simulink model "part1_2"  (R2019b)
settings: Solver=VariableStepAuto  StartTime=0.0  StopTime=9  RelTol=1e-3
libraries: simulink x1
settings Model: Creator=wes_m  LastModifiedBy=wes_m

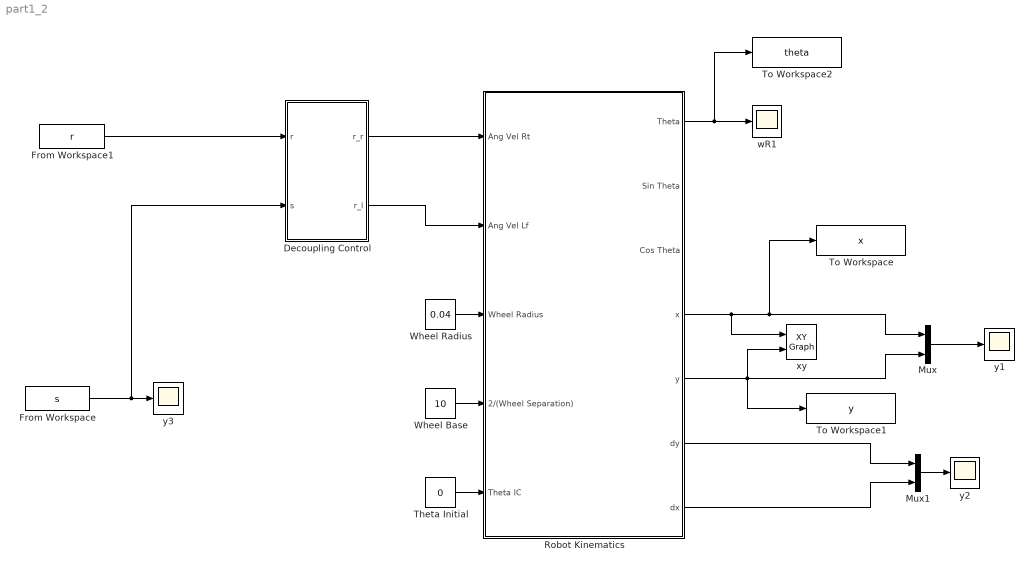
== system part1_2 ==
  Decoupling Control : Subsystem
  From Workspace : FromWorkspace  VariableName=s  SampleTime=0
  From Workspace1 : FromWorkspace  VariableName=r  SampleTime=0
  Mux : Mux  Inputs=2
  Mux1 : Mux  Inputs=2
  Robot Kinematics : Subsystem
  Theta Initial : Constant  Value=0  VectorParams1D=off  OutDataTypeStr=double
  To Workspace : ToWorkspace  VariableName=x  SampleTime=-1
  To Workspace1 : ToWorkspace  VariableName=y  SampleTime=-1
  To Workspace2 : ToWorkspace  VariableName=theta  SampleTime=-1
  Wheel Base : Constant  Value=10
  Wheel Radius : Constant  Value=0.04
  wR1 : Scope
  xy : simulink/Sinks/XY Graph  xmin=-0.1  xmax=0.5  ymin=-0.1  ymax=0.1  st=-1
  y1 : Scope
  y2 : Scope
  y3 : Scope
  wires:
  Decoupling Control/2("r_l ") -> Robot Kinematics/2(Ang Vel Lf)
  From Workspace/1 -> y3/1, Decoupling Control/2(s)
  Mux1/1 -> y2/1
  Robot Kinematics/6(dy) -> Mux1/1
  Theta Initial/1 -> Robot Kinematics/5(Theta IC)
  Decoupling Control/1(r_r) -> Robot Kinematics/1(Ang Vel Rt)
  Robot Kinematics/5(y) -> To Workspace1/1, xy/2, Mux/2
  Wheel Base/1 -> Robot Kinematics/4(2/(Wheel Separation))
  From Workspace1/1 -> Decoupling Control/1(r)
  Robot Kinematics/1(Theta) -> To Workspace2/1, wR1/1
  Robot Kinematics/4(x) -> xy/1, To Workspace/1, Mux/1
  Wheel Radius/1 -> Robot Kinematics/3(Wheel Radius)
  Mux/1 -> y1/1
  Robot Kinematics/7(dx) -> Mux1/2

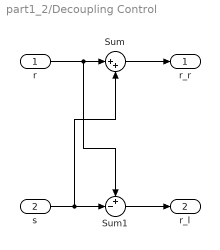
== system part1_2/Decoupling Control ==
  r : Inport
  s : Inport  Port=2
  Sum : Sum  Inputs=|++
  Sum1 : Sum  Inputs=+-|
  r_r : Outport
  "r_l " : Outport  Port=2
  wires:
  Sum1/1 -> "r_l "/1
  s/1 -> Sum/2, Sum1/2
  r/1 -> Sum1/1, Sum/1
  Sum/1 -> r_r/1

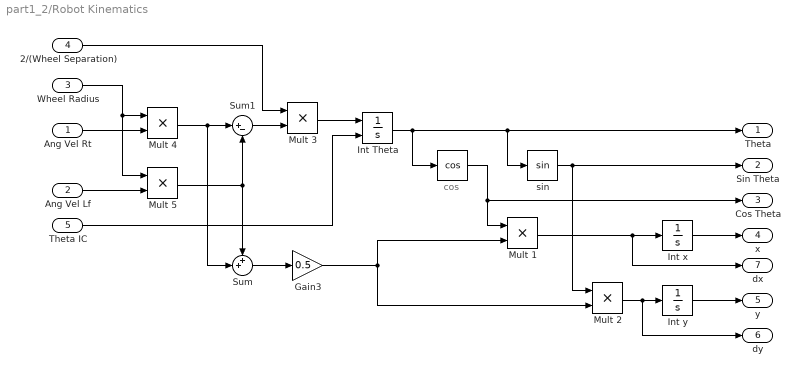
== system part1_2/Robot Kinematics ==
  note: cos
  Ang Vel Rt : Inport
  Ang Vel Lf : Inport  Port=2
  Wheel Radius : Inport  Port=3
  2/(Wheel Separation) : Inport  Port=4
  Theta IC : Inport  Port=5
  " " : Trigonometry  Operator=cos
  Gain3 : Gain  Gain=0.5
  Int Theta : Integrator  InitialConditionSource=external  InitialCondition=1  ZeroCross=off
  Int x : Integrator
  Int y : Integrator
  Mult {1..5} (5 alike) : Product  RndMeth=Zero
  Sum : Sum  Inputs=++|
  Sum1 : Sum  Inputs=|+-
  sin : Trigonometry
  Theta : Outport  VectorParamsAs1DForOutWhenUnconnected=off
  Sin Theta : Outport  Port=2  VectorParamsAs1DForOutWhenUnconnected=off
  Cos Theta : Outport  Port=3  VectorParamsAs1DForOutWhenUnconnected=off
  x : Outport  Port=4  VectorParamsAs1DForOutWhenUnconnected=off
  y : Outport  Port=5  VectorParamsAs1DForOutWhenUnconnected=off
  dy : Outport  Port=6  VectorParamsAs1DForOutWhenUnconnected=off
  dx : Outport  Port=7  VectorParamsAs1DForOutWhenUnconnected=off
  wires:
  Mult 4/1 -> Sum1/1, Sum/2
  Mult 5/1 -> Sum1/2, Sum/1
  Sum1/1 -> Mult 3/2
  Sum/1 -> Gain3/1
  Int Theta/1 -> " "/1, sin/1, Theta/1
  Gain3/1 -> Mult 1/2, Mult 2/2
  " "/1 -> Mult 1/1, Cos Theta/1
  Mult 1/1 -> Int x/1, dx/1
  Mult 2/1 -> Int y/1, dy/1
  sin/1 -> Mult 2/1, Sin Theta/1
  Int x/1 -> x/1
  Int y/1 -> y/1
  Mult 3/1 -> Int Theta/1
  Ang Vel Lf/1 -> Mult 5/2
  Ang Vel Rt/1 -> Mult 4/2
  Wheel Radius/1 -> Mult 4/1, Mult 5/1
  2/(Wheel Separation)/1 -> Mult 3/1
  Theta IC/1 -> Int Theta/2
